simulink model "model_for_figure"  (R2016b)
settings: Solver=VariableStepAuto  StartTime=0.0  StopTime=5000  RelTol=1e-3
values from neighbouring files (symbols this model uses):
  omega = 0.6    [coba_journal.m]    (also in main.m)
undefined symbols (not defined in the file or in its folder): sigbuilder_block
settings Model: Creator=utomo  LastModifiedBy=utomo

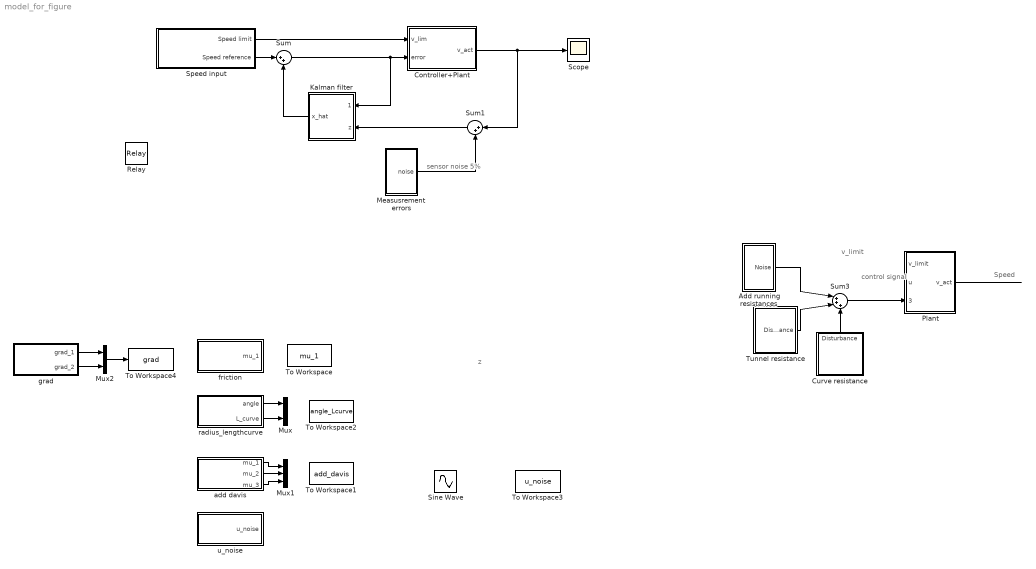
== system model_for_figure ==
  note: Speed
  note: control
      | signal
  note: v_limit
  note: sensor noise
      | 5%
  note: z
  Add running resistances : Subsystem
  Controller+Plant : Subsystem
  Curve resistance : Subsystem
  Kalman filter : Subsystem
  Measusrement errors : Subsystem
  Mux : Mux  Inputs=2
  Mux1 : Mux  Inputs=3
  Mux2 : Mux  Inputs=2
  Plant : Subsystem
  Relay : Relay
  Scope : Scope
  Sine Wave : Sin  Amplitude=1e-5^2  Frequency=1/100  SampleTime=1
  Speed input : Subsystem  Tag=STV Subsys  LoadFcn=sigbuilder_block('load');  StartFcn=sigbuilder_block('start');  StopFcn=sigbuilder_block('stop');  ClipboardFcn=sigbuilder_block('clipboard');  mask(Sigbuilder block){tuvar=[0:10]}
      mask help: Simulink:masks:SigbuilderBlock_MD
      mask init:
      | if ~strcmp(get_param(bdroot(gcbh),'SimulationStatus'),'stopped') tuvar = sigbuilder_block('maskInit'); end
      settings: CopyFcn=sigbuilder_block('copy');  DeleteFcn=sigbuilder_block('delete');  ModelCloseFcn=sigbuilder_block('modelClose');  PreSaveFcn=sigbuilder_block('preSave');  PauseFcn=sigbuilder_block('pause');  ContinueFcn=sigbuilder_block('continue');  NameChangeFcn=sigbuilder_block('namechange');  OpenFcn=sigbuilder_block('open',[437.25 153 550.5 359.25 ]);  CloseFcn=sigbuilder_block('close');
      mask Display: plot(0, 0, 100, 100,[2, 2, 32, 32, 2], [68, 8, 8, 68, 68],[32, 2], [38, 38], [32, 19, 2],[53, 60, 44], [32, 17, 17, 2],[16, 16, 31, 31]);txt = getActiveGroup(gcbh);text(2, 100, txt,'verticalAlignment', 'top');
  Sum : Sum  Inputs=|++
  Sum1 : Sum  Inputs=|++
  Sum3 : Sum  Inputs=|+++
  To Workspace : ToWorkspace  VariableName=mu_1  SampleTime=1
      settings: Save2DSignal=2-D array (concatenate along first dimension)
  To Workspace1 : ToWorkspace  VariableName=add_davis  SampleTime=1
      settings: Save2DSignal=2-D array (concatenate along first dimension)
  To Workspace2 : ToWorkspace  VariableName=angle_Lcurve  SampleTime=1
      settings: Save2DSignal=2-D array (concatenate along first dimension)
  To Workspace3 : ToWorkspace  VariableName=u_noise  SampleTime=1
      settings: Save2DSignal=2-D array (concatenate along first dimension)
  To Workspace4 : ToWorkspace  VariableName=grad  SampleTime=1
      settings: Save2DSignal=2-D array (concatenate along first dimension)
  Tunnel resistance : Subsystem
  add davis : Subsystem  Tag=STV Subsys  LoadFcn=sigbuilder_block('load');  StartFcn=sigbuilder_block('start');  StopFcn=sigbuilder_block('stop');  ClipboardFcn=sigbuilder_block('clipboard');  mask(Sigbuilder block){tuvar=[0:10]}
      mask help: Simulink:masks:SigbuilderBlock_MD
      mask init:
      | if ~strcmp(get_param(bdroot(gcbh),'SimulationStatus'),'stopped') tuvar = sigbuilder_block('maskInit'); end
      settings: CopyFcn=sigbuilder_block('copy');  DeleteFcn=sigbuilder_block('delete');  ModelCloseFcn=sigbuilder_block('modelClose');  PreSaveFcn=sigbuilder_block('preSave');  PauseFcn=sigbuilder_block('pause');  ContinueFcn=sigbuilder_block('continue');  NameChangeFcn=sigbuilder_block('namechange');  OpenFcn=sigbuilder_block('open',[437.25 153 550.5 359.25 ]);  CloseFcn=sigbuilder_block('close');
      mask Display: plot(0, 0, 100, 100,[2, 2, 32, 32, 2], [68, 8, 8, 68, 68],[32, 2], [38, 38], [32, 19, 2],[53, 60, 44], [32, 17, 17, 2],[16, 16, 31, 31]);txt = getActiveGroup(gcbh);text(2, 100, txt,'verticalAlignment', 'top');
  "friction " : Subsystem  Tag=STV Subsys  LoadFcn=sigbuilder_block('load');  StartFcn=sigbuilder_block('start');  StopFcn=sigbuilder_block('stop');  ClipboardFcn=sigbuilder_block('clipboard');  mask(Sigbuilder block){tuvar=[0:10]}
      mask help: Simulink:masks:SigbuilderBlock_MD
      mask init:
      | if ~strcmp(get_param(bdroot(gcbh),'SimulationStatus'),'stopped') tuvar = sigbuilder_block('maskInit'); end
      settings: CopyFcn=sigbuilder_block('copy');  DeleteFcn=sigbuilder_block('delete');  ModelCloseFcn=sigbuilder_block('modelClose');  PreSaveFcn=sigbuilder_block('preSave');  PauseFcn=sigbuilder_block('pause');  ContinueFcn=sigbuilder_block('continue');  NameChangeFcn=sigbuilder_block('namechange');  OpenFcn=sigbuilder_block('open',[437.25 153 550.5 359.25 ]);  CloseFcn=sigbuilder_block('close');
      mask Display: plot(0, 0, 100, 100,[2, 2, 32, 32, 2], [68, 8, 8, 68, 68],[32, 2], [38, 38], [32, 19, 2],[53, 60, 44], [32, 17, 17, 2],[16, 16, 31, 31]);txt = getActiveGroup(gcbh);text(2, 100, txt,'verticalAlignment', 'top');
  grad : Subsystem  Tag=STV Subsys  LoadFcn=sigbuilder_block('load');  StartFcn=sigbuilder_block('start');  StopFcn=sigbuilder_block('stop');  ClipboardFcn=sigbuilder_block('clipboard');  mask(Sigbuilder block){tuvar=[0:10]}
      mask help: Simulink:masks:SigbuilderBlock_MD
      mask init:
      | if ~strcmp(get_param(bdroot(gcbh),'SimulationStatus'),'stopped') tuvar = sigbuilder_block('maskInit'); end
      settings: CopyFcn=sigbuilder_block('copy');  DeleteFcn=sigbuilder_block('delete');  ModelCloseFcn=sigbuilder_block('modelClose');  PreSaveFcn=sigbuilder_block('preSave');  PauseFcn=sigbuilder_block('pause');  ContinueFcn=sigbuilder_block('continue');  NameChangeFcn=sigbuilder_block('namechange');  OpenFcn=sigbuilder_block('open',[437.25 153 550.5 359.25 ]);  CloseFcn=sigbuilder_block('close');
      mask Display: plot(0, 0, 100, 100,[2, 2, 32, 32, 2], [68, 8, 8, 68, 68],[32, 2], [38, 38], [32, 19, 2],[53, 60, 44], [32, 17, 17, 2],[16, 16, 31, 31]);txt = getActiveGroup(gcbh);text(2, 100, txt,'verticalAlignment', 'top');
  radius_lengthcurve : Subsystem  Tag=STV Subsys  LoadFcn=sigbuilder_block('load');  StartFcn=sigbuilder_block('start');  StopFcn=sigbuilder_block('stop');  ClipboardFcn=sigbuilder_block('clipboard');  mask(Sigbuilder block){tuvar=[0:10]}
      mask help: Simulink:masks:SigbuilderBlock_MD
      mask init:
      | if ~strcmp(get_param(bdroot(gcbh),'SimulationStatus'),'stopped') tuvar = sigbuilder_block('maskInit'); end
      settings: CopyFcn=sigbuilder_block('copy');  DeleteFcn=sigbuilder_block('delete');  ModelCloseFcn=sigbuilder_block('modelClose');  PreSaveFcn=sigbuilder_block('preSave');  PauseFcn=sigbuilder_block('pause');  ContinueFcn=sigbuilder_block('continue');  NameChangeFcn=sigbuilder_block('namechange');  OpenFcn=sigbuilder_block('open',[416.25 111.75 550.5 359.25 ]);  CloseFcn=sigbuilder_block('close');
      mask Display: plot(0, 0, 100, 100,[2, 2, 32, 32, 2], [68, 8, 8, 68, 68],[32, 2], [38, 38], [32, 19, 2],[53, 60, 44], [32, 17, 17, 2],[16, 16, 31, 31]);txt = getActiveGroup(gcbh);text(2, 100, txt,'verticalAlignment', 'top');
  u_noise : Subsystem  Tag=STV Subsys  LoadFcn=sigbuilder_block('load');  StartFcn=sigbuilder_block('start');  StopFcn=sigbuilder_block('stop');  ClipboardFcn=sigbuilder_block('clipboard');  mask(Sigbuilder block){tuvar=[0:10]}
      mask help: Simulink:masks:SigbuilderBlock_MD
      mask init:
      | if ~strcmp(get_param(bdroot(gcbh),'SimulationStatus'),'stopped') tuvar = sigbuilder_block('maskInit'); end
      settings: CopyFcn=sigbuilder_block('copy');  DeleteFcn=sigbuilder_block('delete');  ModelCloseFcn=sigbuilder_block('modelClose');  PreSaveFcn=sigbuilder_block('preSave');  PauseFcn=sigbuilder_block('pause');  ContinueFcn=sigbuilder_block('continue');  NameChangeFcn=sigbuilder_block('namechange');  OpenFcn=sigbuilder_block('open',[437.25 153 550.5 359.25 ]);  CloseFcn=sigbuilder_block('close');
      mask Display: plot(0, 0, 100, 100,[2, 2, 32, 32, 2], [68, 8, 8, 68, 68],[32, 2], [38, 38], [32, 19, 2],[53, 60, 44], [32, 17, 17, 2],[16, 16, 31, 31]);txt = getActiveGroup(gcbh);text(2, 100, txt,'verticalAlignment', 'top');
  wires:
  Speed input/2(Speed reference) -> Sum/1
  Measusrement errors/1(noise) -> Sum1/2
  Sum1/1 -> Kalman filter/2(z)
  Kalman filter/1(x_hat) -> Sum/2
  radius_lengthcurve/1(angle) -> Mux/1
  radius_lengthcurve/2(L_curve) -> Mux/2
  add davis/2(mu_2) -> Mux1/2
  add davis/3(mu_3) -> Mux1/3
  add davis/1(mu_1) -> Mux1/1
  Sum3/1 -> Plant/3(disturbances)
  Add running resistances/1(Noise) -> Sum3/1
  Tunnel resistance/1(Disturbance) -> Sum3/2
  Curve resistance/1(Disturbance) -> Sum3/3
  ? -> Plant/1(v_limit)
  ? -> Plant/2(u)
  Plant/1(v_act) -> ?
  grad/1(grad_1) -> Mux2/1
  grad/2(grad_2) -> Mux2/2
  Mux2/1 -> To Workspace4/1
  Controller+Plant/1(v_act) -> Scope/1, Sum1/1
  Speed input/1(Speed limit) -> Controller+Plant/1(v_lim)
  Sum/1 -> Kalman filter/1(sys_in), Controller+Plant/2(error)

== system model_for_figure/Add running resistances ==
  Gain : Gain
  Noise : Outport
  wires:
  ? -> Gain/1
  Gain/1 -> Noise/1

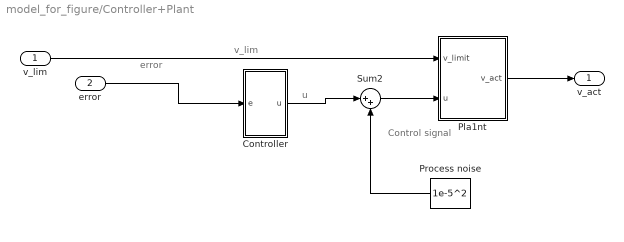
== system model_for_figure/Controller+Plant ==
  note: error
  note: v_lim
  note: Control
      | signal
  note: u
  v_lim : Inport
  error : Inport  Port=2
  Controller : Subsystem
  Pla1nt : Subsystem
  Process noise : Constant  Value=1e-5^2
  Sum2 : Sum  Inputs=|++
  v_act : Outport
  wires:
  error/1 -> Controller/1(e)
  Controller/1(u) -> Sum2/1
  v_lim/1 -> Pla1nt/1(v_limit)
  Pla1nt/1(v_act) -> v_act/1
  Sum2/1 -> Pla1nt/2(u)
  Process noise/1 -> Sum2/2

== system model_for_figure/Curve resistance ==
  Gain : Gain
  Disturbance : Outport
  wires:
  ? -> Gain/1
  Gain/1 -> Disturbance/1

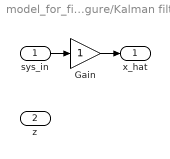
== system model_for_figure/Kalman filter ==
  sys_in : Inport
  z : Inport  Port=2
  Gain : Gain
  x_hat : Outport
  wires:
  sys_in/1 -> Gain/1
  Gain/1 -> x_hat/1

== system model_for_figure/Measusrement errors ==
  Gain : Gain
  noise : Outport
  wires:
  Gain/1 -> noise/1
  ? -> Gain/1

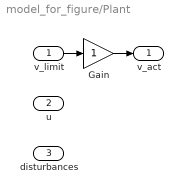
== system model_for_figure/Plant ==
  v_limit : Inport
  u : Inport  Port=2
  disturbances : Inport  Port=3
  Gain : Gain
  v_act : Outport
  wires:
  Gain/1 -> v_act/1
  v_limit/1 -> Gain/1

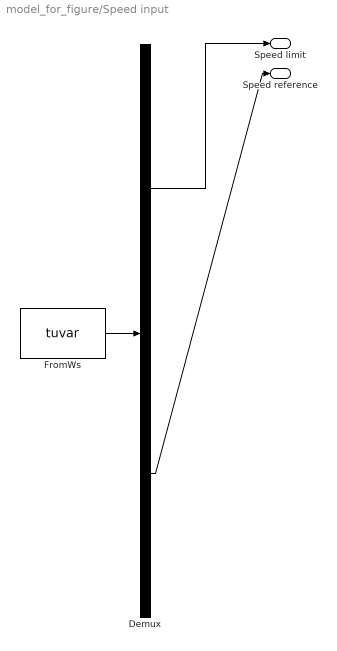
== system model_for_figure/Speed input ==
  Demux : Demux  Tag=STV Demux  Outputs=2
  FromWs : FromWorkspace  Tag=STV FromWs  VariableName=tuvar  SampleTime=0
      SigBuilderData=|
      | common.afterFinalStr = 'Extrapolate'
      | common.sampleTime = 0
      | dataSet.timeRange = [0 10]
      | dataSet.name = 'Group 1'
      | sbobj.Groups.Name = 'Group 1'
      | sbobj.Groups.Signals(1).Name = 'Speed limit'
      | sbobj.Groups.Signals(1).XData = [0 4 4 6 6 10]
      | sbobj.Groups.Signals(1).YData = [0 0 1 1 0 0]
      | sbobj.Groups.Signals(2).Name = 'Speed reference'
      | sbobj.Groups.Signals(2).XData = [0 10]
      | sbobj.Groups.Signals(2).YData = [0 0]
  Speed limit : Outport  Tag=STV Outport
  Speed reference : Outport  Tag=STV Outport  Port=2
  wires:
  Demux/1 -> Speed limit/1
  FromWs/1 -> Demux/1
  Demux/2 -> Speed reference/1

== system model_for_figure/Tunnel resistance ==
  Gain : Gain
  Disturbance : Outport
  wires:
  Gain/1 -> Disturbance/1
  ? -> Gain/1

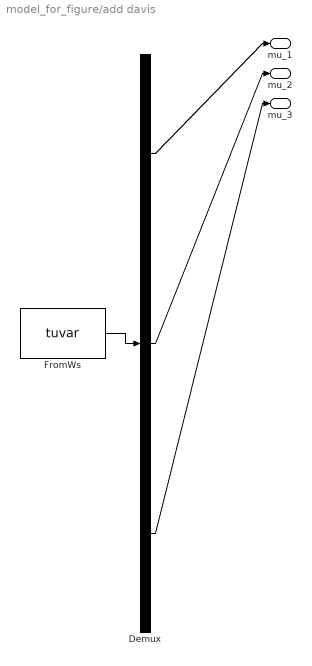
== system model_for_figure/add davis ==
  Demux : Demux  Tag=STV Demux  Outputs=3
  FromWs : FromWorkspace  Tag=STV FromWs  VariableName=tuvar
      SigBuilderData=|
      | common.afterFinalStr = 'Extrapolate'
      | common.sampleTime = '-1'
      | dataSet.timeRange = [0 5000]
      | dataSet.name = 'Group 1'
      | sbobj.Groups.Name = 'Group 1'
      | sbobj.Groups.Signals(1).Name = 'mu_1'
      | sbobj.Groups.Signals(1).XData = [0 500 500 1000 1500 2000 2000 2500 3000 3500 4000 4500 5000]
      | sbobj.Groups.Signals(1).YData = [1 0.7 0.9 1.1 1 1.2 0.8 0.9 0.9 1.1 1.05 0.9 1.1]
      | sbobj.Groups.Signals(2).Name = 'mu_2'
      | sbobj.Groups.Signals(2).XData = [0 500 500 1000 1500 2000 2000 2500 3000 3500 4000 4500 5000]
      | sbobj.Groups.Signals(2).YData = [0.9 1 0.9 1 0.8 1 1.1 0.7 1.2 0.9 1 1.1 0.9]
      | sbobj.Groups.Signals(3).Name = 'mu_3'
      | sbobj.Groups.Signals(3).XData = [0 500 500 1000 1500 2000 2000 2500 3000 3500 4000 4500 5000]
      | sbobj.Groups.Signals(3).YData = [0.7 0.8 1 0.8 1.1 0.8 1 1.05 1.1 1.2 0.8 0.9 0.99]
      | sbobj.Groups.TimeRange = [0 5000]
  mu_1 : Outport  Tag=STV Outport
  mu_2 : Outport  Tag=STV Outport  Port=2
  mu_3 : Outport  Tag=STV Outport  Port=3
  wires:
  Demux/1 -> mu_1/1
  FromWs/1 -> Demux/1
  Demux/2 -> mu_2/1
  Demux/3 -> mu_3/1

== system model_for_figure/friction  ==
  Demux : Demux  Tag=STV Demux  Outputs=1
  FromWs : FromWorkspace  Tag=STV FromWs  VariableName=tuvar
      SigBuilderData=|
      | common.afterFinalStr = 'Extrapolate'
      | common.sampleTime = '-1'
      | dataSet.timeRange = [0 5000]
      | dataSet.name = 'Group 1'
      | sbobj.Groups.Name = 'Group 1'
      | sbobj.Groups.Signals.Name = 'mu_1'
      | sbobj.Groups.Signals.XData = [0 3.24 500 1000 1500 2000 2000 2500 3000 3500 4000 4500 5000]
      | sbobj.Groups.Signals.YData = [0 0 0.1 0.385 0.6 0.25 0.05 0.305 0.9 0.8 0.7 0.2 0.499401197605]
      | sbobj.Groups.TimeRange = [0 5000]
  mu_1 : Outport  Tag=STV Outport
  wires:
  FromWs/1 -> Demux/1
  Demux/1 -> mu_1/1

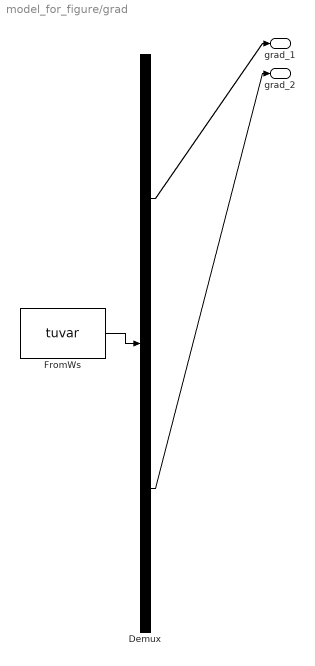
== system model_for_figure/grad ==
  Demux : Demux  Tag=STV Demux  Outputs=2
  FromWs : FromWorkspace  Tag=STV FromWs  VariableName=tuvar
      SigBuilderData=|
      | common.afterFinalStr = 'Extrapolate'
      | common.sampleTime = '-1'
      | dataSet.timeRange = [0 5000]
      | dataSet.name = 'Group 1'
      | sbobj.Groups.Name = 'Group 1'
      | sbobj.Groups.Signals(1).Name = 'grad_1'
      | sbobj.Groups.Signals(1).XData = [0 3.24 200 400 600 800 1000 1200 1400 1600 1800 1800 2000 2200 2400 2600 2800 3000 3200 3400 3600 3800 4000 4200 4400 4600 4800 5000]
      | sbobj.Groups.Signals(1).YData = [0 0 0.36 2 -2 0.37 1 -3 0.6 2.5 0.48 2 0.31 -1.5 0.175 0.5 -1.8 0.64 3 0.1 1 -1 0.7 1.2 -0.5 -1.5 0.46 0.2]
      | sbobj.Groups.Signals(2).Name = 'grad_2'
      | sbobj.Groups.Signals(2).XData = [0 100 200 400 600 800 1000 1200 1400 1600 1800 1800 2000 2200 2400 2600 2800 3000 3200 3400 3600 3800 4000 4200 4400 4600 4800 5000]
      | sbobj.Groups.Signals(2).YData = [-0.5 0.5 -1 0.2 3 0.37 2 2.8 0.5 -2.5 -2 -1 1.31 1.5 1.75 -3 -2.8 -2.6 -2 2.5 2 2.8 2.5 0 0 0.5 -0.5 -1]
      | sbobj.Groups.TimeRange = [0 5000]
  grad_1 : Outport  Tag=STV Outport
  grad_2 : Outport  Tag=STV Outport  Port=2
  wires:
  Demux/1 -> grad_1/1
  FromWs/1 -> Demux/1
  Demux/2 -> grad_2/1

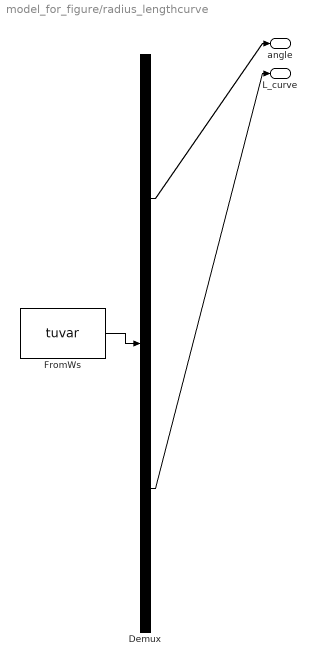
== system model_for_figure/radius_lengthcurve ==
  Demux : Demux  Tag=STV Demux  Outputs=2
  FromWs : FromWorkspace  Tag=STV FromWs  VariableName=tuvar
      SigBuilderData=|
      | common.afterFinalStr = 'Extrapolate'
      | common.sampleTime = '-1'
      | dataSet.timeRange = [0 5000]
      | dataSet.name = 'Group 1'
      | sbobj.Groups.Name = 'Group 1'
      | sbobj.Groups.Signals(1).Name = 'angle'
      | sbobj.Groups.Signals(1).XData = [0 3.24 101 101 300 300 3001 3001 4000 4000 4401 4401 4900 4900 5000]
      | sbobj.Groups.Signals(1).YData = [0 0 0 90 90 0 0 190 190 0 0 75 75 0 0]
      | sbobj.Groups.Signals(2).Name = 'L_curve'
      | sbobj.Groups.Signals(2).XData = [0 3.24 101 101 300 300 3001 3001 4000 4000 4401 4401 4900 4900 5000]
      | sbobj.Groups.Signals(2).YData = [0 0 0 200 200 0 0 1000 1000 0 0 500 500 0 0]
      | sbobj.Groups.TimeRange = [0 5000]
  angle : Outport  Tag=STV Outport
  L_curve : Outport  Tag=STV Outport  Port=2
  wires:
  Demux/1 -> angle/1
  FromWs/1 -> Demux/1
  Demux/2 -> L_curve/1

== system model_for_figure/u_noise ==
  Demux : Demux  Tag=STV Demux  Outputs=1
  FromWs : FromWorkspace  Tag=STV FromWs  VariableName=tuvar
      SigBuilderData=|
      | common.afterFinalStr = 'Extrapolate'
      | common.sampleTime = '-1'
      | dataSet.timeRange = [0 5000]
      | dataSet.name = 'Group 1'
      | sbobj.Groups.Name = 'Group 1'
      | sbobj.Groups.Signals.Name = 'u_noise'
      | sbobj.Groups.Signals.XData = [0 500 500 1000 1000 1500 1500 2000 2000 2500 2500 3000 3000 3500 3500 4000 4000 4500 4500 5000]
      | sbobj.Groups.Signals.YData = [0 1e-10 0 -1e-10 0 1e-10 0 -1e-10 0 1e-10 0 -1e-10 0 1e-10 0 -1e-10 0 1e-10 0 -1e-10]
      | sbobj.Groups.TimeRange = [0 5000]
  u_noise : Outport  Tag=STV Outport
  wires:
  Demux/1 -> u_noise/1
  FromWs/1 -> Demux/1

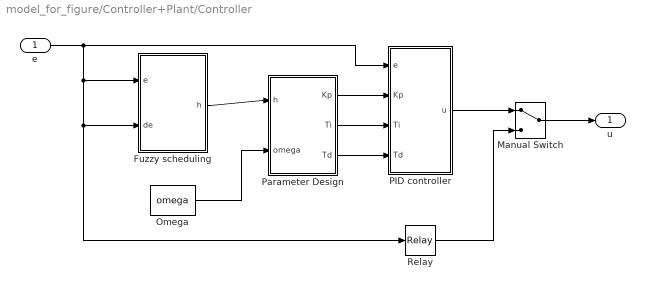
== system model_for_figure/Controller+Plant/Controller ==
  e : Inport
  Fuzzy scheduling : Subsystem
  Manual Switch : ManualSwitch
  Omega : Constant  Value=omega
  PID controller : Subsystem
  Parameter Design : Subsystem
  Relay : Relay
  u : Outport
  wires:
  e/1 -> Relay/1, Fuzzy scheduling/2(de), Fuzzy scheduling/1(e), PID controller/1(e)
  PID controller/1(u) -> Manual Switch/1
  Relay/1 -> Manual Switch/2
  Fuzzy scheduling/1(h) -> Parameter Design/1(h)
  Omega/1 -> Parameter Design/2(omega)
  Parameter Design/2(Ti) -> PID controller/3(Ti)
  Parameter Design/1(Kp) -> PID controller/2(Kp)
  Parameter Design/3(Td) -> PID controller/4(Td)
  Manual Switch/1 -> u/1

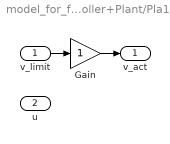
== system model_for_figure/Controller+Plant/Pla1nt ==
  v_limit : Inport
  u : Inport  Port=2
  Gain : Gain
  v_act : Outport
  wires:
  v_limit/1 -> Gain/1
  Gain/1 -> v_act/1

== system model_for_figure/Controller+Plant/Controller/Fuzzy scheduling ==
  e : Inport
  de : Inport  Port=2
  Gain : Gain
  h : Outport
  wires:
  Gain/1 -> h/1

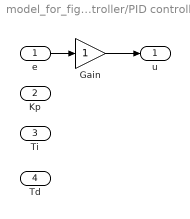
== system model_for_figure/Controller+Plant/Controller/PID controller ==
  e : Inport
  Kp : Inport  Port=2
  Ti : Inport  Port=3
  Td : Inport  Port=4
  Gain : Gain
  u : Outport
  wires:
  Gain/1 -> u/1
  e/1 -> Gain/1

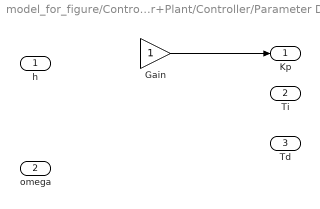
== system model_for_figure/Controller+Plant/Controller/Parameter Design ==
  h : Inport
  omega : Inport  Port=2
  Gain : Gain
  Kp : Outport
  Ti : Outport  Port=2
  Td : Outport  Port=3
  wires:
  Gain/1 -> Kp/1
